simulink model "sim_1"  (R2024b)
settings: Solver=VariableStepAuto  StartTime=0.0  StopTime=total_time  RelTol=1e-3
undefined symbols (not defined in the file): control_par, controller_index, D, d_actual, d_nom, kf, ki, P_INIT_EKF, prob_gps_loss, qf, qi, R_2, R_3, R_4, R_5, r_actual, r_nom, Ta, Tc, total_time, Ts, w_max, X, Y, Z_INIT_EKF
libraries: robotlib x4
settings Model: Creator=riccardo01  LastModifiedBy=leontecosm

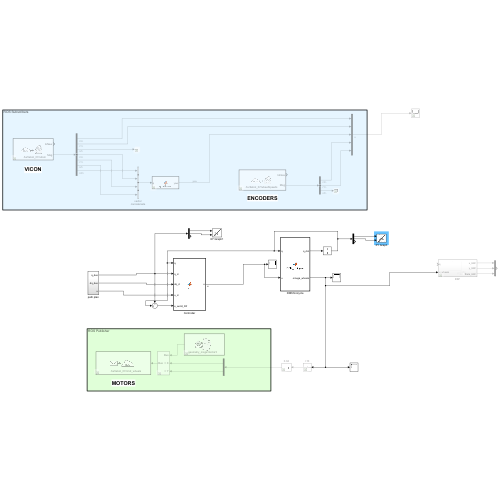
[thumbnail: Simulink's stored preview of the top-level diagram]
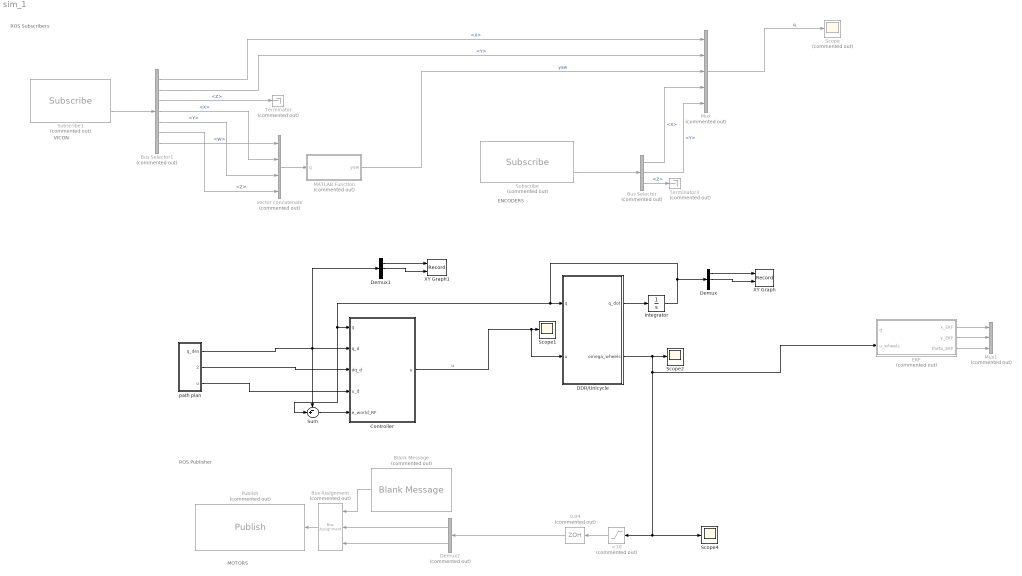
== system sim_1 ==
  note: MOTORS
  note: ROS Publisher
  note: ENCODERS
  note: VICON
  note: ROS Subscribers
  0.04 : ZeroOrderHold  Commented=on  SampleTime=Ts
  <10 : Saturate  Commented=on  UpperLimit=w_max  LowerLimit=-w_max
  Blank Message : robotlib/Blank Message  Commented=on  messageClass=Message  entityType=geometry_msgs/Vector3  messageType=geometry_msgs/Vector3  SampleTime=Ts  legacyBusStruct=off
      settings: LibrarySourceBlock=roslib/ROS/Blank Message
  Bus Assignment : BusAssignment  Commented=on  AssignedSignals=X,Y
  Bus Selector : BusSelector  Commented=on  OutputSignals=X,Y,Z
  Bus Selector1 : BusSelector  Commented=on  OutputSignals=Pose.Pose.Position.X,Pose.Pose.Position.Y,Pose.Pose.Position.Z,Pose.Pose.Orientation.X,Pose.Pose.Orientation.Y,Pose.Pose.Orientation.Z,Pose.Pose.Orientation.W
  Controller : MATLAB Function  TreatAsAtomicUnit=on
  DDR/Unicycle : MATLAB Function  TreatAsAtomicUnit=on
  Demux : Demux  Outputs=3
  Demux1 : Demux  Outputs=3
  Demux2 : Demux  Commented=on  Outputs=2
  EKF : Subsystem  Commented=on
  Integrator : Integrator  InitialCondition=qi
  MATLAB Function : MATLAB Function  Commented=on  TreatAsAtomicUnit=on
  Mux : Mux  Commented=on  Inputs=5
  Mux1 : Mux  Commented=on  Inputs=3
  Publish : robotlib/Publish  Commented=on  topicSource=Specify your own  topic=/turtlebot_07/cmd_wheels  messageType=geometry_msgs/Vector3  legacyBusStruct=off  messageQueueLength=1
      settings: LibrarySourceBlock=roslib/ROS/Publish
  Scope : Scope  Commented=on
  Scope1 : Scope
  Scope2 : Scope
  Scope4 : Scope
  Subscribe : robotlib/Subscribe  Commented=on  topicSource=Specify your own  topic=/turtlebot_07/wheelSpeeds  messageType=geometry_msgs/Vector3  SampleTime=-1  legacyBusStruct=off  messageQueueLength=1
      settings: LibrarySourceBlock=roslib/ROS/Subscribe
  Subscribe1 : robotlib/Subscribe  Commented=on  topicSource=Specify your own  topic=/turtlebot_07/odom  messageType=nav_msgs/Odometry  SampleTime=-1  legacyBusStruct=off  messageQueueLength=1
      settings: LibrarySourceBlock=roslib/ROS/Subscribe
  Sum : Sum  Inputs=-+|
  Terminator : Terminator  Commented=on
  Terminator3 : Terminator  Commented=on
  XY Graph : Record  FileSettingsInternal="{\"entries\":[{\"content\":{\"excelSettings\":{\"content\":{},\"type\":\"Streamout.ExcelSettings\"}},\"type\":\"Streamout.FileSettingStorage\",\"uuid\":\"\"}],\"packageUris\":[\"http:\\/\\/schema.mathworks.com\\/mf0\\/streamout_blocks\\/R2020a\"],\"version\":\"1.0\"}"  Layout=[1 1]  SignalsInternal="{\"entries\":[{\"content\":{\"signals\":[{\"content\":{\"blockPath\":[],\"dimensions\":[1,1],\"domain\":\"\",\"lineColor\":\"#a2142f\",\"plots\":[ 1 ],\"port\":1,\"sid\":[\"\"],\"signalID\":1,\"signalName\":\"Demux:1\"},\"type\":\"RecordBlkView.Signal\",\"uuid\":\"\"},{\"content\":{\"blockPath\":[],\"dimensions\":[1,1],\"domain\":\"\",\"lineColor\":\"#139fff\",\"plots\":[ 1 ],\"port\":2,\"sid\":[\"\"],\"signalID\":2,\"signalName\":\"Demux:2\"},\"type\":\"RecordBlkView.Signal\",\"uuid\":\"\"}]},\"type\":\"RecordBlkView.InputSignals\",\"uuid\":\"\"}],\"packageUris\":[\"http:\\/\\/schema.mathworks.com\\/mf0\\/streamout_blocks\\/R2020a\"],\"version\":\"1.0\"}"  VisualizationBindings="{\"xyplotplugin\":{\"info\":[{\"series\":[{\"bindingParametersList\":[{\"parameter\":\"X-Axis\",\"signalID\":1,\"signalName\":\"Demux:1\"},{\"parameter\":\"Y-Axis\",\"signalID\":2,\"signalName\":\"Demux:2\"}],\"seriesID\":0}],\"subplotID\":1}]}}"  CompatibilityTag=XY
  XY Graph1 : Record  FileSettingsInternal="{\"entries\":[{\"content\":{\"excelSettings\":{\"content\":{},\"type\":\"Streamout.ExcelSettings\"}},\"type\":\"Streamout.FileSettingStorage\",\"uuid\":\"\"}],\"packageUris\":[\"http:\\/\\/schema.mathworks.com\\/mf0\\/streamout_blocks\\/R2020a\"],\"version\":\"1.0\"}"  Layout=[1 1]  SignalsInternal="{\"entries\":[{\"content\":{\"signals\":[{\"content\":{\"blockPath\":[],\"dimensions\":[1,1],\"domain\":\"\",\"lineColor\":\"#a2142f\",\"plots\":[ 1 ],\"port\":1,\"sid\":[\"\"],\"signalID\":1,\"signalName\":\"Demux1:1\"},\"type\":\"RecordBlkView.Signal\",\"uuid\":\"\"},{\"content\":{\"blockPath\":[],\"dimensions\":[1,1],\"domain\":\"\",\"lineColor\":\"#139fff\",\"plots\":[ 1 ],\"port\":2,\"sid\":[\"\"],\"signalID\":2,\"signalName\":\"Demux1:2\"},\"type\":\"RecordBlkView.Signal\",\"uuid\":\"\"}]},\"type\":\"RecordBlkView.InputSignals\",\"uuid\":\"\"}],\"packageUris\":[\"http:\\/\\/schema.mathworks.com\\/mf0\\/streamout_blocks\\/R2020a\"],\"version\":\"1.0\"}"  VisualizationBindings="{\"xyplotplugin\":{\"info\":[{\"series\":[{\"bindingParametersList\":[{\"parameter\":\"X-Axis\",\"signalID\":1,\"signalName\":\"Demux1:1\"},{\"parameter\":\"Y-Axis\",\"signalID\":2,\"signalName\":\"Demux1:2\"}],\"seriesID\":0}],\"subplotID\":1}]}}"  CompatibilityTag=XY
  path plan : Subsystem
  vector concatenate : Concatenate  Commented=on  NumInputs=4
  wires:
  0.04/1 -> Demux2/1
  Blank Message/1 -> Bus Assignment/1
  <10/1 -> 0.04/1
  Demux2/2 -> Bus Assignment/3
  Bus Assignment/1 -> Publish/1
  Demux2/1 -> Bus Assignment/2
  DDR/Unicycle/2(omega_wheels) -> <10/1, Scope4/1, EKF/2(u_wheels), Scope2/1
  vector concatenate/1 -> MATLAB Function/1(q)
  Subscribe/2 -> Bus Selector/1
  Bus Selector1/5 -> vector concatenate/3  "<Y>"
  Bus Selector/2 -> Mux/5  "<Y>"
  Bus Selector1/3 -> Terminator/1  "<Z>"
  Bus Selector1/1 -> Mux/1  "<X>"
  MATLAB Function/1(yaw) -> Mux/3  "yaw"
  Subscribe1/2 -> Bus Selector1/1
  Bus Selector1/6 -> vector concatenate/4  "<Z>"
  Bus Selector/1 -> Mux/4  "<X>"
  Mux/1 -> Scope/1  "q"
  Bus Selector/3 -> Terminator3/1  "<Z>"
  Bus Selector1/2 -> Mux/2  "<Y>"
  Bus Selector1/7 -> vector concatenate/1  "<W>"
  Bus Selector1/4 -> vector concatenate/2  "<X>"
  EKF/2(y_EKF) -> Mux1/2
  EKF/1(x_EKF) -> Mux1/1
  EKF/3(theta_EKF) -> Mux1/3
  path plan/2(dq_des) -> Controller/3(dq_d)
  path plan/3(u) -> Controller/4(u_d)
  Sum/1 -> Controller/5(e_world_RF)
  Controller/1(u) -> Scope1/1, DDR/Unicycle/2(u)  "u"
  DDR/Unicycle/1(q_dot) -> Integrator/1
  Integrator/1 -> Demux/1, Sum/2, Controller/1(q), DDR/Unicycle/1(q)
  Demux/1 -> XY Graph/1
  Demux/2 -> XY Graph/2
  path plan/1(q_des) -> Controller/2(q_d), Sum/1, Demux1/1
  Demux1/1 -> XY Graph1/1
  Demux1/2 -> XY Graph1/2

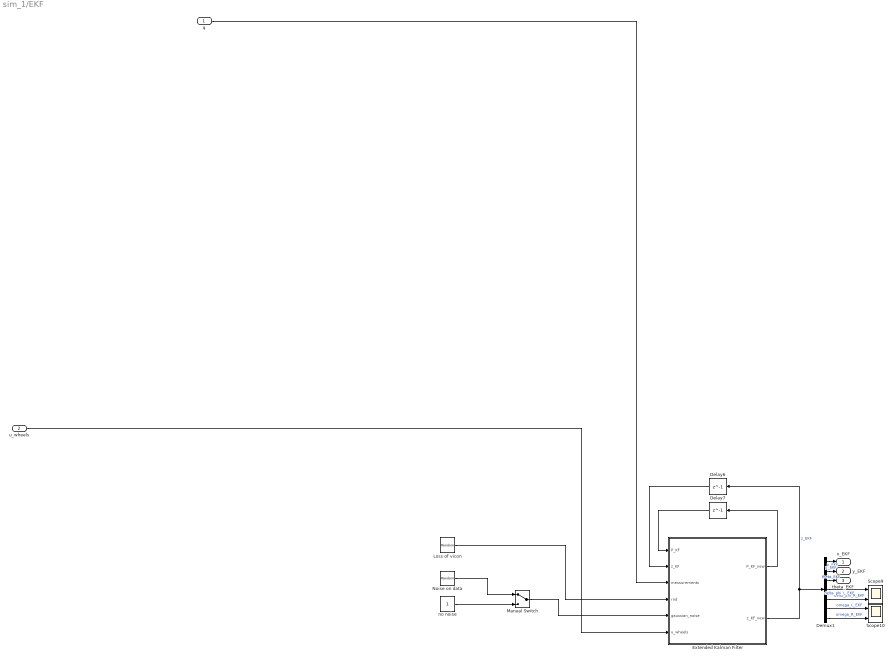
== system sim_1/EKF ==
  q : Inport
  u_wheels : Inport  Port=2
  " Loss of vicon" : UniformRandomNumber  Minimum=0
  Delay6 : Delay  DelayLength=1  InitialCondition=Z_INIT_EKF
  Delay7 : Delay  DelayLength=1  InitialCondition=P_INIT_EKF
  Demux1 : Demux  Outputs=7
  Extended Kalman Filter : MATLAB Function  TreatAsAtomicUnit=on
  Manual Switch : ManualSwitch
  Noise on data : RandomNumber  Variance=0.0001
  Scope10 : Scope  NumInputPorts=2
  Scope9 : Scope  NumInputPorts=2
  no noise : Constant
  x_EKF : Outport
  y_EKF : Outport  Port=2
  theta_EKF : Outport  Port=3
  wires:
  Demux1/6 -> Scope10/1  "omega_L_EKF"
  Demux1/3 -> theta_EKF/1  "theta_EKF"
  Delay6/1 -> Extended Kalman Filter/2(z_KF)
  Delay7/1 -> Extended Kalman Filter/1(P_KF)
  Noise on data/1 -> Manual Switch/1
  Demux1/5 -> Scope9/2  "delta_phi_R_EKF"
  Demux1/7 -> Scope10/2  "omega_R_EKF"
  Extended Kalman Filter/1(P_KF_new) -> Delay7/1
  Manual Switch/1 -> Extended Kalman Filter/5(gaussian_noise)
  " Loss of vicon"/1 -> Extended Kalman Filter/4(rnd)
  Demux1/1 -> x_EKF/1  "x_EKF"
  Demux1/4 -> Scope9/1  "delta_phi_L_EKF"
  no noise/1 -> Manual Switch/2
  u_wheels/1 -> Extended Kalman Filter/6(u_wheels)
  Extended Kalman Filter/2(z_KF_new) -> Demux1/1, Delay6/1  "z_EKF"
  q/1 -> Extended Kalman Filter/3(messurements)
  Demux1/2 -> y_EKF/1  "y_EKF"

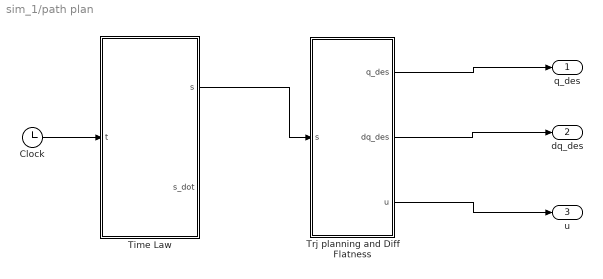
== system sim_1/path plan ==
  Clock : Clock
      settings: Decimation=1/Ts
  Time Law : MATLAB Function  TreatAsAtomicUnit=on
  Trj planning and Diff Flatness : MATLAB Function  TreatAsAtomicUnit=on
  q_des : Outport
  dq_des : Outport  Port=2
  u : Outport  Port=3
  wires:
  Clock/1 -> Time Law/1(t)
  Time Law/1(s) -> Trj planning and Diff Flatness/1(s)
  Trj planning and Diff Flatness/1(q_des) -> q_des/1
  Trj planning and Diff Flatness/3(u) -> u/1
  Trj planning and Diff Flatness/2(dq_des) -> dq_des/1

== matlab function sim_1/Controller ==
  data: q input; q_d input; dq_d input; u_d input; u output; e_world_RF input; controller_index parameter; control_par parameter
function u = fcn(q, q_d, dq_d, u_d, e_world_RF, controller_index, control_par)
% compute the error in the unicycle RF
M=[ cos(q(3)),  sin(q(3)),  0;
    -sin(q(3)), cos(q(3)),  0;
    0,               0,       1];
e=M*e_world_RF;

e(3)=wrapToPi(e(3));

if controller_index == 1
    % linear controller
    %control_par = [xi, a, 0];
    
    k3 = 2*control_par(1)*control_par(2);
    k1 = k3;
    k2 = (control_par(2)^2 - u_d(2)^2)/u_d(1);
    u = [k1*e(1) + cos(e(3))*u_d(1); 
        k2*e(2)+k3*e(3) + u_d(2)];

    

elseif controller_index == 2
    % nonlinear controller
    %control_par = [xi, b, 0];
    %singularity avoidance
    if e(3)<=10^-3 && e(3)>=-10^-3
        e(3)=10^-3;
    end

    k2 = control_par(2);
    
    k1 = 2*control_par(1)*sqrt(u_d(1)*control_par(2) + u_d(2)^2);
    k3 = k1;

    u = [k1*e(1)+ cos(e(3))*u_d(1);
        k2*(u_d(1)*sin(e(3))/e(3))*e(2) + k3*e(3)+ u_d(2)];



elseif controller_index == 3
    % feedback linearization
    %control_par = [k1, k2,b];
    k1=control_par(1);
    k2=control_par(2);
    b=control_par(3);

    v=u_d(1);
    w=u_d(2);

    %evaluation b point
    Xb=q(1)+b*cos(q(3));
    Yb=q(2)+b*sin(q(3));

    %evaluation b point desired
    Xb_d=q_d(1)+b*cos(q(3));
    Yb_d=q_d(2)+b*sin(q(3));

    %evaluation derivatives b point desired
    dXb_d=dq_d(1)-b*sin(q(3))*dq_d(3);
    dYb_d=dq_d(2)+b*cos(q(3))*dq_d(3);

    %matrix b poit to point
    T_inv=[ cos(q(3)),      sin(q(3));
            -sin(q(3))/b,   cos(q(3))/b];

    %evaluation of controll law
    u = T_inv*[ dXb_d+k1*(Xb_d-Xb);
                dYb_d+k2*(Yb_d-Yb)];
else
    u = u_d;
end

== matlab function sim_1/DDR//Unicycle ==
  data: q_dot output; q input; u input; omega_wheels output; d_nom parameter; r_nom parameter; w_max parameter
function [q_dot,omega_wheels]  = DDR_Unicycle(q, u, d_nom, r_nom,w_max)
v = u(1);
omega = u(2);
omega_M = w_max;

q_dot = [cos(q(3))*v; sin(q(3))*v; omega];

%evaluation of speed wheels
omega_l = (2*v - d_nom*omega) / (2*r_nom);
omega_r = (2*v + d_nom*omega) / (2*r_nom);

% if (abs(omega_l)>=omega_M)||(abs(omega_r)>=omega_M)%if atleast one of the weel is in saturation
%     W_m=max([abs(omega_l),abs(omega_r)]);
% 
%     omega_l=(omega_l/W_m)*omega_M;
%     omega_r=(omega_r/W_m)*omega_M;
% end

omega_wheels = [omega_l;omega_r];

== matlab function sim_1/path plan/Time Law ==
  data: t input; s output; s_dot output; total_time parameter; Ta parameter; Tc parameter
function [s, s_dot] = fcn(t,total_time,Ta, Tc)
s=0;
s_dot=0;

Vc=1/(Ta+Tc);% velocità costante
a=Vc/Ta;% acceleration

switch 1 %formula on the slide
    case t<Ta
        s_dot=a*t;
        s=(a*(t^2))/2;

    case (t>=Ta)&&(t<(Tc+Ta))
        s_dot=Vc;
        s=(a*(Ta^2))/2+Vc*(t-Ta);

    case (t>=(Tc+Ta))&&(t<(Tc+2*Ta))
        s_dot=Vc-a*(t-Ta-Tc);
        s=(a*(Ta^2))/2+Vc*Tc+Vc*(t-Ta-Tc)-a*(t-Ta-Tc)^2/2;

    case t>=(Tc+2*Ta)
        s_dot=0;
        s=1;


end

== matlab function sim_1/path plan/Trj planning and Diff Flatness ==
  data: q_des output; dq_des output; qi parameter; qf parameter; s input; u output; ki parameter; kf parameter
function [q_des,dq_des,u]  =Path_planning_cartesian(qi, qf, s, ki, kf)
    % s as vector like 0:0.1:1000
    %evaluate the weight as written in the slide
    a1 = qf(1);
    a2 = qi(1);
    b1 = qf(2);
    b2 = qi(2);
    
    a4 = ki*cos(qi(3)) + 3*qi(1);
    a3 = kf*cos(qf(3)) - 3*qf(1);
    
    b4 = ki*sin(qi(3)) + 3*qi(2);
    b3 = kf*sin(qf(3)) - 3*qf(2);
    
    % evaluate path
    x = a1*s.^3 - a2*(s-1).^3 + a3*s.^2.*(s-1) + a4*s.*(s-1).^2;
    y = b1*s.^3 - b2*(s-1).^3 + b3*s.^2.*(s-1) + b4*s.*(s-1).^2;

    %analitical calculation of velocity
    x_dot=3*a1*s.^2-3*a2*(s-1).^2+a3*(2*s.*(s-1)+s.^2)+a4*((s-1).^2+s.*2.*(s-1));
    y_dot=3*b1*s.^2-3*b2*(s-1).^2+b3*(2*s.*(s-1)+s.^2)+b4*((s-1).^2+s.*2.*(s-1));

    %analitical calculation of acceleration
    x_ddot=6*a1*s-6*a2*(s-1)+a3*(2*s+2*(s+(s-1)))+a4*(2*(s-1)+2*((s-1)+s));
    y_ddot=6*b1*s-6*b2*(s-1)+b3*(2*s+2*(s+(s-1)))+b4*(2*(s-1)+2*((s-1)+s));
    
    theta = atan2(y_dot, x_dot);
    q_des = [x, y,theta]';
    
    v = sqrt(y_dot^2 +  x_dot^2);
    omega = (x_dot*y_ddot - y_dot*x_ddot)/(y_dot^2 +  x_dot^2);

    dq_des = [x_dot,y_dot,omega]';
    u = [v,omega]';

end

== matlab function sim_1/EKF/Extended Kalman Filter ==
  data: P_KF input; P_KF_new output; z_KF input; messurements input; D parameter; R_2 parameter; R_3 parameter; R_4 parameter; R_5 parameter; r_actual parameter; d_actual parameter; rnd input; gaussian_noise input; z_KF_new output; u_wheels input; Ts parameter; prob_gps_loss parameter
function [P_KF_new, z_KF_new] = EKF_filtering(P_KF, z_KF, messurements, D, R_2, R_3, R_4, R_5 ,r_actual, d_actual, rnd, gaussian_noise,u_wheels, Ts,prob_gps_loss)

% z_KF = [x_EKF, y_EKF, theta_EKF, delta_phi_L_EKF, delta_phi_R_EKF, omega_L_EKF, omega_R_EKF]

v_k = r_actual * (z_KF(6) + z_KF(7))/2;
w_k = r_actual * (z_KF(7) - z_KF(6))/d_actual;

theta_mean = z_KF(3) + (w_k * Ts)/2;

F_k = [1, 0, -Ts * v_k * sin(theta_mean), 0, 0, Ts * r_actual * cos(theta_mean)/2 + (Ts)^2 * r_actual * v_k * sin(theta_mean)/(2*d_actual), Ts * r_actual * cos(theta_mean)/2 - (Ts)^2 * r_actual * v_k * sin(theta_mean)/(2*d_actual);
    0, 1, Ts * v_k * cos(theta_mean), 0, 0, Ts * r_actual * sin(theta_mean)/2 - (Ts)^2 * r_actual * v_k * cos(theta_mean)/(2*d_actual), Ts * r_actual * sin(theta_mean)/2 + (Ts)^2 * r_actual * v_k * cos(theta_mean)/(2*d_actual);
    0, 0, 1, 0, 0, (-Ts*r_actual)/d_actual, (Ts*r_actual)/d_actual;
    0, 0, 0, 0, 0, Ts, 0;
    0, 0, 0, 0, 0, 0, Ts;
    0, 0, 0, 0, 0, 0, 0;
    0, 0, 0, 0, 0, 0, 0];

%% Prediction part

z_pred = [z_KF(1)+(Ts*r_actual*(z_KF(6)+z_KF(7))/2)*cos(theta_mean + (Ts*r_actual*(z_KF(6)+z_KF(7)))/(2*d_actual));
    z_KF(2)+(Ts*r_actual*(z_KF(6)+z_KF(7))/2)*sin(theta_mean + (Ts*r_actual*(z_KF(7)-z_KF(6)))/(2*d_actual));
    theta_mean + (Ts*r_actual*(z_KF(7)-z_KF(6))/(2*d_actual));
    Ts*z_KF(6);
    Ts*z_KF(7);
    u_wheels(1);
    u_wheels(2)];

P_pred = F_k * P_KF * F_k' + D;


%% Update
messurements = [messurements;u_wheels];
if(rnd<prob_gps_loss) 

    % Just encoders
    y_messurement = [messurements(1); messurements(2)];
    H = [0, 0, 0, 1, 0, 0, 0;
        0, 0, 0, 0, 1, 0, 0];

    e = y_messurement - H * z_pred;
    K = P_pred * H' /(H * P_pred * H' + R_2);

    z_KF_new = z_pred +  K * e;
    P_KF_new = P_pred - K * H * P_pred;

else 
    % GPS(x,y,yaw) + Encoders(omegaL,omegaR)
    y_messurement = [messurements(1)+gaussian_noise;messurements(2)+gaussian_noise; messurements(3)+gaussian_noise;messurements(4); messurements(5)];

    H = [1, 0, 0, 0, 0, 0, 0;
         0, 1, 0, 0, 0, 0, 0;
         0, 0, 1, 0, 0, 0, 0;
         0, 0, 0, 0, 0, 1, 0;
         0, 0, 0, 0, 0, 0, 1];

    e = y_messurement - H * z_pred;
    K = P_pred * H' /(H * P_pred * H' + R_5);

    z_KF_new = z_pred + K * e;
    P_KF_new = P_pred - K * H * P_pred;

end

== matlab function sim_1/MATLAB Function ==
  data: q input; yaw output
function yaw = quat2yaw(q)

% normalize to avoid issues
q = q / norm(q);

w = q(1);
x = q(2);
y = q(3);
z = q(4);

% rotation around Z axis
yaw = atan2(2*(w*z + x*y), 1 - 2*(y^2 + z^2));

end
